simulink model "Final_Longitudinal__"  (R2022a)
settings: Solver=VariableStepAuto  StartTime=0.0  StopTime=20  MinStep=0.001  RelTol=1e-6  AbsTol=1e-6
values from neighbouring files (symbols this model uses):
  AL = [-0.83705 1.7696 -0.35236 0; -5.9575 -21.766 0.0056738 0.8717; 0 0 0 1; 14.891 -47.637 -0.015802 -7.9269]    [Longitudinal_parameters.m]
  BL = [0 3.9397; -0.91092 0; 0 0; -30.902 -6.9048]    [Longitudinal_parameters.m]
  KL = [KL_hat(:,1) KL_hat(:,2) KL_hat(:,3) KL_hat(:,4)]    [Longitudinal_parameters.m]
  kli = [KL_hat(:,5) KL_hat(:,6)]    [Longitudinal_parameters.m]
libraries: dspsrcs4 x1
settings Model: Creator=Lenovo  LastModifiedBy=ankit
settings SolverCC: InitialStep=0.01
settings DebuggingCC: UnconnectedInputMsg=warning  UnconnectedOutputMsg=warning  UnconnectedLineMsg=warning
settings RTWCC: DLArmComputeVersion=19.05

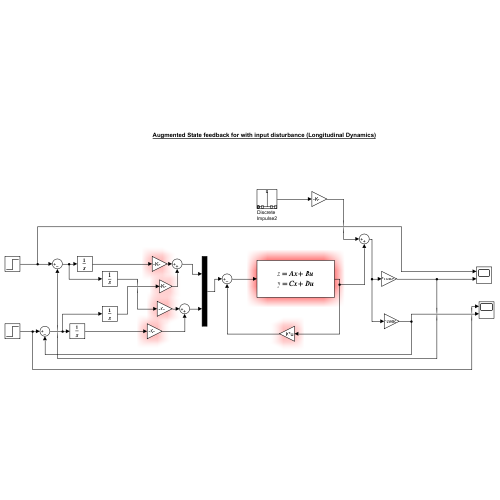
[thumbnail: Simulink's stored preview of the top-level diagram]
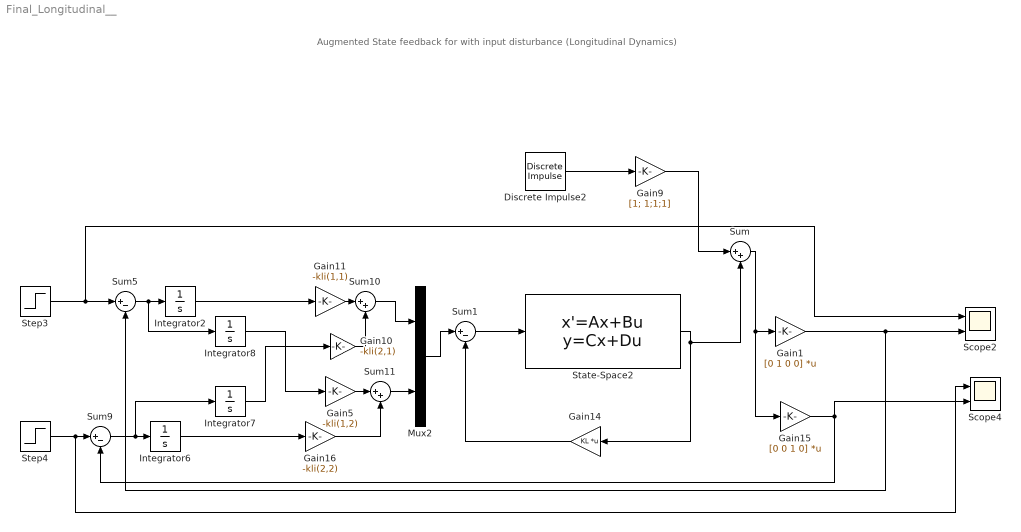
== system Final_Longitudinal__ ==
  note: Augmented State feedback for with input disturbance (Longitudinal Dynamics)
  Discrete Impulse2 : dspsrcs4/Discrete  Impulse  Delay=0  SampleTime=1  FrameSample=1  OutputFrames=off  dataType=double  isSigned=on  wordLen=16  udDataType=sfix(16)  fracBitsMode=Best precision  numFracBits=15  OutDataTypeStr=double  LastOutDataTypeStr=double
  Gain1 : Gain  Gain=[0 1 0 0]  Multiplication=Matrix(K*u) (u vector)
  Gain10 : Gain  Gain=-kli(2,1)
  Gain11 : Gain  Gain=-kli(1,1)
  Gain14 : Gain  Gain=KL  Multiplication=Matrix(K*u)
  Gain15 : Gain  Gain=[0 0 1 0]  Multiplication=Matrix(K*u) (u vector)
  Gain16 : Gain  Gain=-kli(2,2)
  Gain5 : Gain  Gain=-kli(1,2)
  Gain9 : Gain  Gain=[1; 1;1;1]
  Integrator{2,6..8} (4 alike) : Integrator
  Mux2 : Mux  Inputs=2
  Scope2 : Scope  NumInputPorts=2
  Scope4 : Scope  NumInputPorts=2
  State-Space2 : StateSpace  A=AL  B=BL  C=eye(4)  D=zeros(4,2)  InitialCondition=0
  Step3 : Step  Time=0  SampleTime=0
  Step4 : Step  Time=0  SampleTime=0
  Sum : Sum  Inputs=|++
  Sum1 : Sum  Inputs=|+-
  Sum10 : Sum  Inputs=|++
  Sum11 : Sum  Inputs=|++
  Sum5 : Sum  Inputs=|+-
  Sum9 : Sum  Inputs=|+-
  wires:
  Gain16/1 -> Sum11/2
  Gain14/1 -> Sum1/2
  Sum10/1 -> Mux2/1
  Gain15/1 -> Scope4/2, Sum9/2
  Gain5/1 -> Sum11/1
  Integrator2/1 -> Gain11/1
  Integrator7/1 -> Gain10/1
  Gain10/1 -> Sum10/2
  Gain11/1 -> Sum10/1
  Sum11/1 -> Mux2/2
  Gain1/1 -> Scope2/2, Sum5/2
  Integrator8/1 -> Gain5/1
  Integrator6/1 -> Gain16/1
  Sum1/1 -> State-Space2/1
  Step4/1 -> Scope4/1, Sum9/1
  Step3/1 -> Sum5/1, Scope2/1
  Sum5/1 -> Integrator8/1, Integrator2/1
  Mux2/1 -> Sum1/1
  Sum9/1 -> Integrator7/1, Integrator6/1
  Discrete Impulse2/1 -> Gain9/1
  State-Space2/1 -> Sum/2, Gain14/1
  Gain9/1 -> Sum/1
  Sum/1 -> Gain1/1, Gain15/1
